simulink model "PostureRegulator"  (R2024b)
settings: Solver=FixedStepAuto  StartTime=0.0  StopTime=T  FixedStep=Ts  RelTol=1e-3
InitFcn:
  | alpha=1;
  | R=0.2;
  | 
  | qi=[alpha+1,1,pi/4]';
  | qf=[0,0,0]';
  | T=20;
  | Ts=0.001;
  | Tso=0.05;
StopFcn:
  | plotting;
libraries: robotmobilelib x1
settings Model: Creator=salva  LastModifiedBy=salva

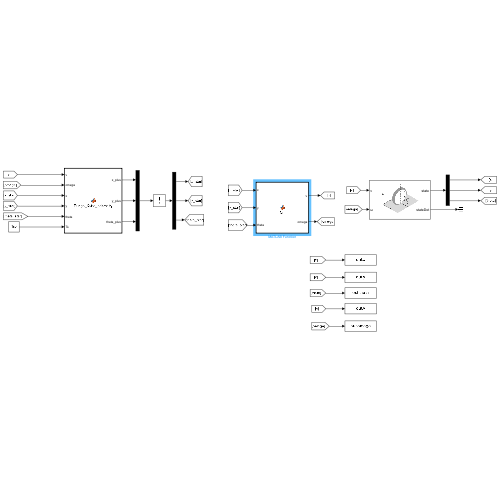
[thumbnail: Simulink's stored preview of the top-level diagram]
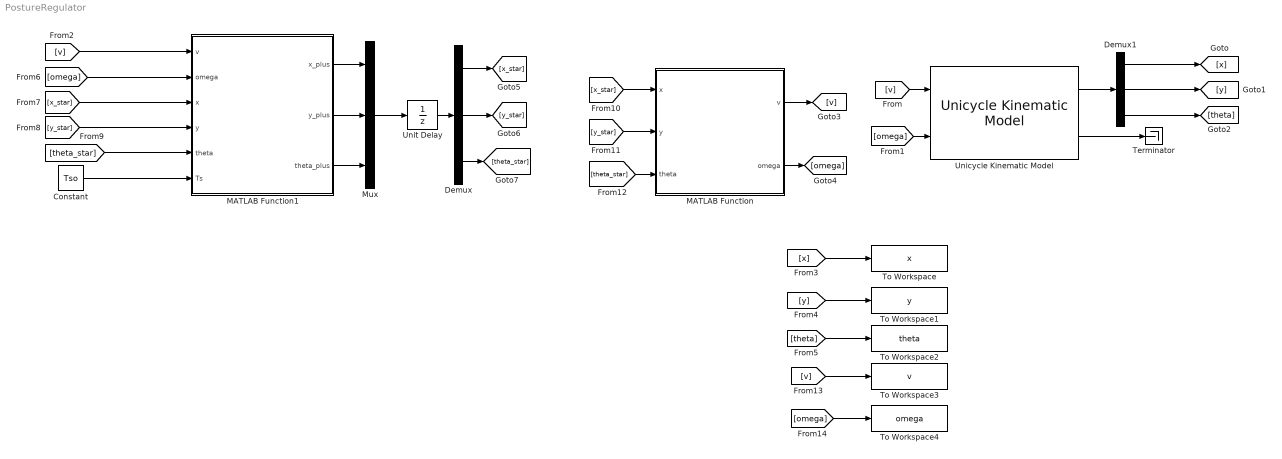
== system PostureRegulator ==
  Constant : Constant  Value=Tso
  Demux : Demux  Outputs=3
  Demux1 : Demux  Outputs=3
  MATLAB Function : MATLAB Function  TreatAsAtomicUnit=on
  MATLAB Function1 : MATLAB Function  TreatAsAtomicUnit=on
  Mux : Mux  Inputs=3
  Terminator : Terminator
  To Workspace : ToWorkspace  VariableName=x  SaveFormat=Timeseries  SampleTime=Ts
  To Workspace1 : ToWorkspace  VariableName=y  SaveFormat=Timeseries  SampleTime=Ts
  To Workspace2 : ToWorkspace  VariableName=theta  SaveFormat=Timeseries  SampleTime=Ts
  To Workspace3 : ToWorkspace  VariableName=v  SaveFormat=Timeseries  SampleTime=Tso
  To Workspace4 : ToWorkspace  VariableName=omega  SaveFormat=Timeseries  SampleTime=Tso
  Unicycle Kinematic Model : robotmobilelib/Unicycle Kinematic Model  VehicleInputs=Vehicle Speed & Heading Angular Velocity  WheelRadius=R  WheelSpeedRange=[-Inf Inf]  InitialState=qi  SimulateUsing=Interpreted execution
  Unit Delay : UnitDelay  InitialCondition=qi  SampleTime=Tso  HasFrameUpgradeWarning=on
  wires:
  Unicycle Kinematic Model/1 -> Demux1/1
  Demux1/2 -> [y]
  Demux1/3 -> [theta]
  Demux1/1 -> [x]
  Constant/1 -> MATLAB Function1/6(Ts)
  MATLAB Function/1(v) -> [v]
  MATLAB Function/2(omega) -> [omega]
  [v] -> Unicycle Kinematic Model/1
  [omega] -> Unicycle Kinematic Model/2
  [x_star] -> MATLAB Function/1(x)
  [y_star] -> MATLAB Function/2(y)
  [theta_star] -> MATLAB Function/3(theta)
  [v] -> MATLAB Function1/1(v)
  [omega] -> MATLAB Function1/2(omega)
  [x_star] -> MATLAB Function1/3(x)
  [y_star] -> MATLAB Function1/4(y)
  [theta_star] -> MATLAB Function1/5(theta)
  Unit Delay/1 -> Demux/1
  Demux/1 -> [x_star]
  Demux/2 -> [y_star]
  Demux/3 -> [theta_star]
  MATLAB Function1/1(x_plus) -> Mux/1
  MATLAB Function1/2(y_plus) -> Mux/2
  MATLAB Function1/3(theta_plus) -> Mux/3
  Mux/1 -> Unit Delay/1
  Unicycle Kinematic Model/2 -> Terminator/1
  [x] -> To Workspace/1
  [y] -> To Workspace1/1
  [theta] -> To Workspace2/1
  [v] -> To Workspace3/1
  [omega] -> To Workspace4/1

== matlab function PostureRegulator/MATLAB Function1 ==
  data: v input; x_plus output; omega input; x input; y input; theta input; Ts input; y_plus output; theta_plus output
function [x_plus,y_plus,theta_plus] = Runge_Kutta_odometry(v,omega,x,y,theta,Ts)
    
    x_plus=x+Ts*v*cos(theta+0.5*omega*Ts);
    y_plus=y+Ts*v*sin(theta+0.5*omega*Ts);
    theta_plus=theta+omega*Ts;

== matlab function PostureRegulator/MATLAB Function ==
  data: x input; v output; y input; theta input; omega output
function [v,omega] = fcn(x,y,theta)

rho=sqrt(x^2+y^2);
gamma=atan2(y,x)-theta+pi;
delta=gamma+theta;


k1=1;
k2=2;
k3=1;


    v=k1*rho*cos(gamma);
    omega=k2*gamma+k1*sin(gamma)*cos(gamma)*(1+k3*delta/gamma);


end
